simulink model "Gerando_Psid_d1Psid_simples"  (R2015a)
settings: Solver=ode4  StartTime=0.0  StopTime=tfinal  FixedStep=dt  RelTol=1e-3
values from neighbouring files (symbols this model uses):
  beta = 0.07    [Trabalho_nSimples.m]
  gama = 0.58    [Trabalho_nSimples.m]
  Psid0 = atan2(d1Yd(1),d1Xd(1))    [Trabalho_nSimples.m]
libraries: simulink_extras x1
settings Model: Creator=joniram  LastModifiedBy=José Oniram
settings DataIOCC: SignalLoggingSaveFormat=ModelDataLogs
settings OptimizationCC: ExpressionDepthLimit=2147483647
settings DebuggingCC: UnderspecifiedInitializationDetection=Classic  MergeDetectMultiDrivingBlocksExec=none  FcnCallInpInsideContextMsg=UseLocalSettings  StateNameClashWarn=warning
settings GRTTargetCC: CombineOutputUpdateFcns=off  GRTInterface=on

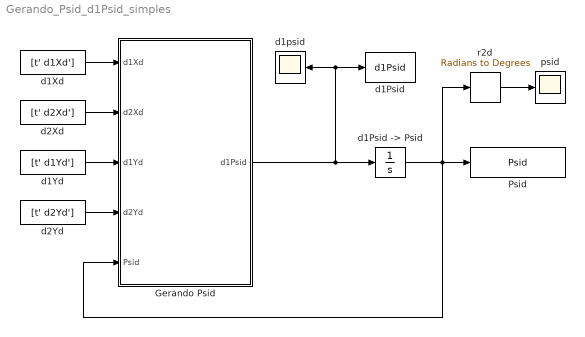
== system Gerando_Psid_d1Psid_simples ==
  "  r2d   " : simulink_extras/Transformations/Radians to Degrees
  Gerando Psid : MATLAB Function  TreatAsAtomicUnit=on
  Psid : ToWorkspace  VariableName=Psid  SampleTime=-1
  d1Psid : ToWorkspace  VariableName=d1Psid  SampleTime=-1
  "d1Psid -> Psid" : Integrator  InitialCondition=Psid0
  d1Xd : FromWorkspace  VariableName=[t' d1Xd']  SampleTime=0  OutputAfterFinalValue=Holding final value
  d1Yd : FromWorkspace  VariableName=[t' d1Yd']  SampleTime=0  OutputAfterFinalValue=Holding final value
  d1psid : Scope
  d2Xd : FromWorkspace  VariableName=[t' d2Xd']  SampleTime=0  OutputAfterFinalValue=Holding final value
  d2Yd : FromWorkspace  VariableName=[t' d2Yd']  SampleTime=0  OutputAfterFinalValue=Holding final value
  psid : Scope
      settings: SaveName=ScopeData5
  wires:
  d1Xd/1 -> Gerando Psid/1(d1Xd)
  d2Xd/1 -> Gerando Psid/2(d2Xd)
  d1Yd/1 -> Gerando Psid/3(d1Yd)
  d2Yd/1 -> Gerando Psid/4(d2Yd)
  Gerando Psid/1(d1Psid) -> "d1Psid -> Psid"/1, d1Psid/1, d1psid/1
  "d1Psid -> Psid"/1 -> Psid/1, "  r2d   "/1, Gerando Psid/5(Psid)
  "  r2d   "/1 -> psid/1

== matlab function Gerando_Psid_d1Psid_simples/Gerando Psid ==
  data: d1Xd input; d2Xd input; d1Psid output; d1Yd input; d2Yd input; gama parameter; beta parameter; Psid input
function d1Psid  = gera_Psid(d1Xd, d2Xd, d1Yd, d2Yd, gama, beta, Psid)

  % Variáveis auxiliares
    aux1 = (d2Xd + beta*d1Xd)*sin(Psid) - (d2Yd + beta*d1Yd)*cos(Psid);
    aux2 = (gama - 1)*(d1Xd*cos(Psid) + d1Yd*sin(Psid));

  % Obtendo d1Psid
    d1Psid = (aux1)/(aux2);
